simulink model "lacroma_main"  (R2023a)
settings: Solver=FixedStepAuto  StartTime=0.0  StopTime=inf  FixedStep=0.05  RelTol=1e-3
libraries: ros2lib x4, MarineRoboticsLib x2, robotcorelib x1
settings Model: Creator=mbat  LastModifiedBy=mbat

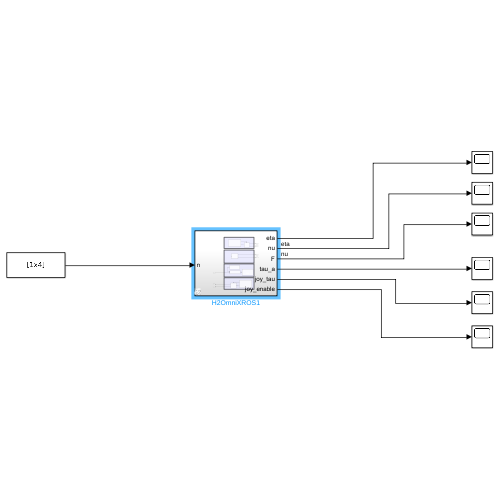
[thumbnail: Simulink's stored preview of the top-level diagram]
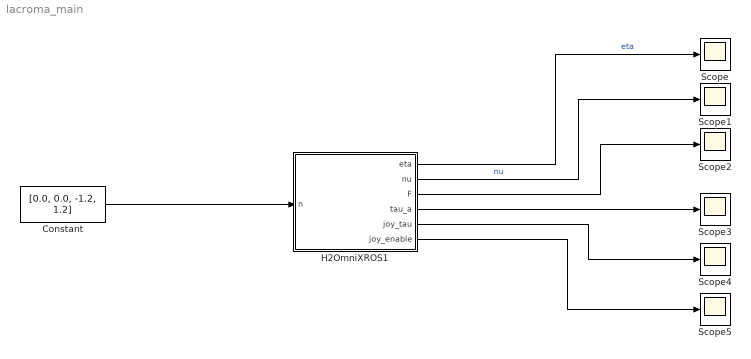
== system lacroma_main ==
  Constant : Constant  Value=[0.0, 0.0, -1.2, 1.2]  OutDataTypeStr=double
  H2OmniXROS1 : Subsystem  AncestorBlock=MarineRoboticsLib/H2OmniXROS1
      settings: LibrarySourceBlock=MarineRoboticsLib/H2OmniXROS1
  Scope{,1..5} (6 alike) : Scope
  wires:
  H2OmniXROS1/1(eta) -> Scope/1  "eta"
  H2OmniXROS1/2(nu) -> Scope1/1  "nu"
  H2OmniXROS1/3(F) -> Scope2/1
  H2OmniXROS1/4(tau_a) -> Scope3/1
  H2OmniXROS1/5(joy_tau) -> Scope4/1
  H2OmniXROS1/6(joy_enable) -> Scope5/1
  Constant/1 -> H2OmniXROS1/1(n)

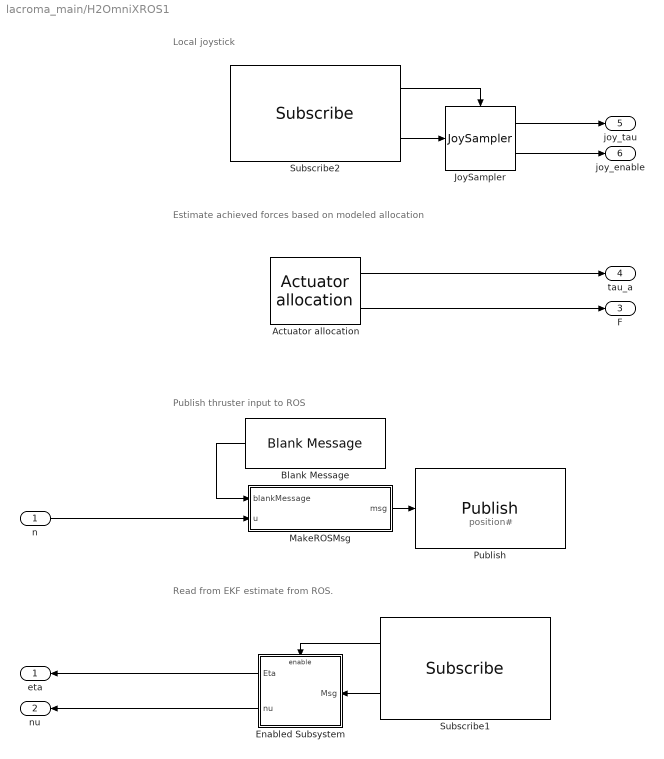
== system lacroma_main/H2OmniXROS1 ==
  note: position#
  note: Local joystick
  note: Read from EKF estimate from ROS.
  note: Publish thruster input to ROS
  note: Estimate achieved forces based on modeled allocation
  n : Inport
  Actuator allocation : MarineRoboticsLib/Actuator allocation  Tm=0  B="[0.25, 0.25, -0.25, -0.25; -0.25,  0.25, -0.25,  0.25; -0.25, 0.25, 0.25, -0.25]"  Keff=[1,1,1,1]
  Blank Message : ros2lib/Blank Message  messageClass=Message  entityType=std_msgs/Float32MultiArray  messageType=std_msgs/Float32MultiArray  SampleTime=0.05
  Enabled Subsystem : Subsystem  TreatAsAtomicUnit=on
  JoySampler : MarineRoboticsLib/JoyOverROS/JoySampler  SystemSampleTime=-1  VariantActivationTime=update diagram  Latency=0  AutoFrameSizeCalculation=off
  MakeROSMsg : MATLAB Function  TreatAsAtomicUnit=on  SystemSampleTime=0.05
  Publish : ros2lib/Publish  topicSource=Specify your own  topic=/lacroma/pwm_out  messageType=std_msgs/Float32MultiArray  QOSHistory=Keep last  QOSDepth=1  QOSReliability=Reliable  QOSDurability=Volatile
  Subscribe1 : ros2lib/Subscribe  topicSource=Specify your own  topic=/lacroma/odometry/filtered  messageType=nav_msgs/Odometry  sampleTime=0.05  QOSHistory=Keep last  QOSDepth=1  QOSReliability=Reliable  QOSDurability=Volatile
  Subscribe2 : ros2lib/Subscribe  topicSource=Specify your own  topic=/lacroma/joy  messageType=sensor_msgs/Joy  sampleTime=0.05  QOSHistory=Keep last  QOSDepth=1  QOSReliability=Reliable  QOSDurability=Volatile
  eta : Outport
  nu : Outport  Port=2
  F : Outport  Port=3
  tau_a : Outport  Port=4
  joy_tau : Outport  Port=5
  joy_enable : Outport  Port=6
  wires:
  n/1 -> MakeROSMsg/2(u)
  MakeROSMsg/1(msg) -> Publish/1
  Subscribe1/2 -> Enabled Subsystem/1(Msg)
  Subscribe1/1 -> Enabled Subsystem/Enable
  Enabled Subsystem/1(Eta) -> eta/1
  Blank Message/1 -> MakeROSMsg/1(blankMessage)
  Enabled Subsystem/2(nu) -> nu/1
  Actuator allocation/2 -> F/1
  Actuator allocation/1 -> tau_a/1
  JoySampler/2 -> joy_enable/1
  Subscribe2/2 -> JoySampler/1
  JoySampler/1 -> joy_tau/1
  Subscribe2/1 -> JoySampler/Enable

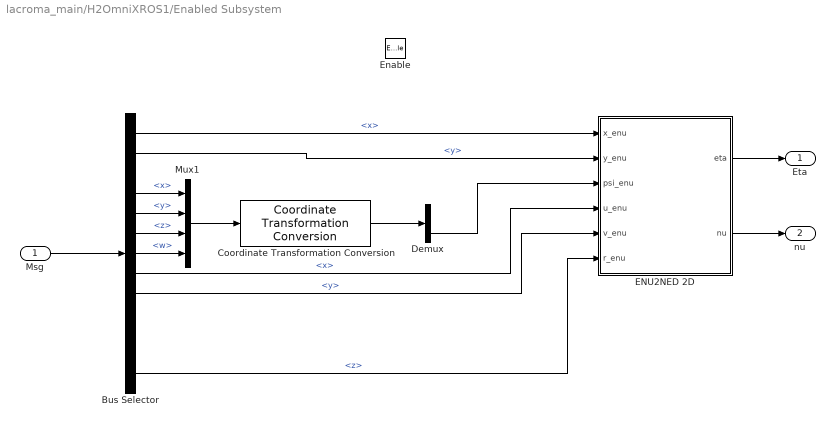
== system lacroma_main/H2OmniXROS1/Enabled Subsystem ==
  Msg : Inport
  Enable : EnablePort
  Bus Selector : BusSelector  OutputSignals=pose.pose.position.x,pose.pose.position.y,pose.pose.position.z,pose.pose.orientation.x,pose.pose.orientation.y,pose.pose.orientation.z,pose.pose.orientation.w,twist.twist.linear.x,twist.twist.linear.y,twist.twist.linear.z,twist.twist.angular.x,twist.twist.angular.y,twist.twist.angular.z
  Coordinate Transformation Conversion : robotcorelib/Coordinate Transformation Conversion  InputRepresentation=Quaternion  InputEulerSequence=ZYX  ShowTrVecInputPort=on  OutputRepresentation=Euler Angles  OutputEulerSequence=ZYX  ShowTrVecOutputPort=on  SimulateUsing=Interpreted execution
      settings: LibrarySourceBlock=roslib/Utilities/Coordinate Transformation Conversion
  Demux : Demux  Outputs=3
  ENU2NED 2D : MATLAB Function  TreatAsAtomicUnit=on
  Mux1 : Mux
  Eta : Outport
  nu : Outport  Port=2
  wires:
  Msg/1 -> Bus Selector/1
  Bus Selector/4 -> Mux1/1  "<x>"
  Bus Selector/5 -> Mux1/2  "<y>"
  Bus Selector/6 -> Mux1/3  "<z>"
  Bus Selector/7 -> Mux1/4  "<w>"
  Mux1/1 -> Coordinate Transformation Conversion/1
  Bus Selector/2 -> ENU2NED 2D/2(y_enu)  "<y>"
  Bus Selector/1 -> ENU2NED 2D/1(x_enu)  "<x>"
  Coordinate Transformation Conversion/1 -> Demux/1
  Bus Selector/8 -> ENU2NED 2D/4(u_enu)  "<x>"
  Bus Selector/9 -> ENU2NED 2D/5(v_enu)  "<y>"
  Bus Selector/13 -> ENU2NED 2D/6(r_enu)  "<z>"
  ENU2NED 2D/1(eta) -> Eta/1
  ENU2NED 2D/2(nu) -> nu/1
  Demux/3 -> ENU2NED 2D/3(psi_enu)

== matlab function lacroma_main/H2OmniXROS1/Enabled Subsystem/ENU2NED 2D ==
  data: x_enu input; eta output; y_enu input; psi_enu input; u_enu input; v_enu input; r_enu input; nu output
function [eta, nu] = enu2ned2d(x_enu,y_enu,psi_enu,u_enu,v_enu,r_enu)
% Just do coordinate swap
psi_ned = pi/2-psi_enu;

psi_ned = mod(psi_ned, 2*pi);

if psi_ned > pi
   psi_ned = -2*pi + psi_ned;
elseif psi_ned <= -pi 
   psi_ned = 2*pi + psi_ned;
end


eta = [y_enu; x_enu; psi_ned];
nu = [u_enu; -v_enu; -r_enu;];

== matlab function lacroma_main/H2OmniXROS1/MakeROSMsg ==
  data: blankMessage input; u input; msg output Bus: SL_Bus_std_msgs_Float32MultiArray
function msg  = assign_bus(blankMessage,u)

% blank message input
msg = blankMessage;

% assign pwm values into data field
msg.data(1:numel(u)) = reshape(u,[],2);

% all other fields must be assigned to complete the message
msg.data_SL_Info.CurrentLength = uint32(numel(u));
msg.layout.dim(1).size = uint32(size(u,1));
msg.layout.dim(2).size = uint32(size(u,2));
msg.layout.dim(1).stride = uint32(numel(u));
msg.layout.dim(2).stride = uint32(prod(size(u,2)));
